simulink model "SC_TestModel"  (R2022b)
settings: Solver=VariableStepAuto  StartTime=0.0  StopTime=SimTime  RelTol=1e-3
undefined symbols (not defined in the file or in its folder): R_bal, SC_nm, SC_np, SC_ns, SC_rc, SC_rv
libraries: spsCurrentMeasurementLib x2, spsSeriesRLCBranchLib x2, spsSupercapacitorLib x1, sps_lib x1
settings Model: Creator=xuupp  LastModifiedBy=xuupp
settings DataIOCC: ReturnWorkspaceOutputs=off

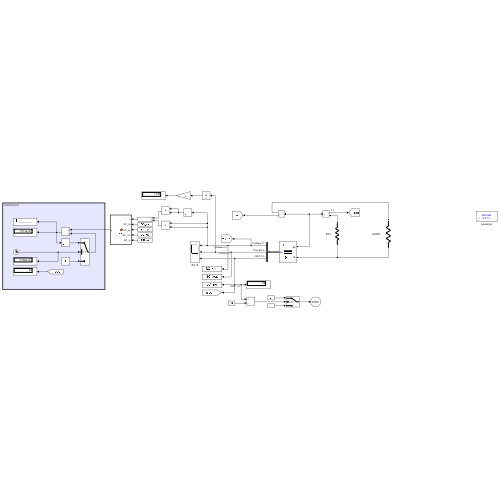
[thumbnail: Simulink's stored preview of the top-level diagram]
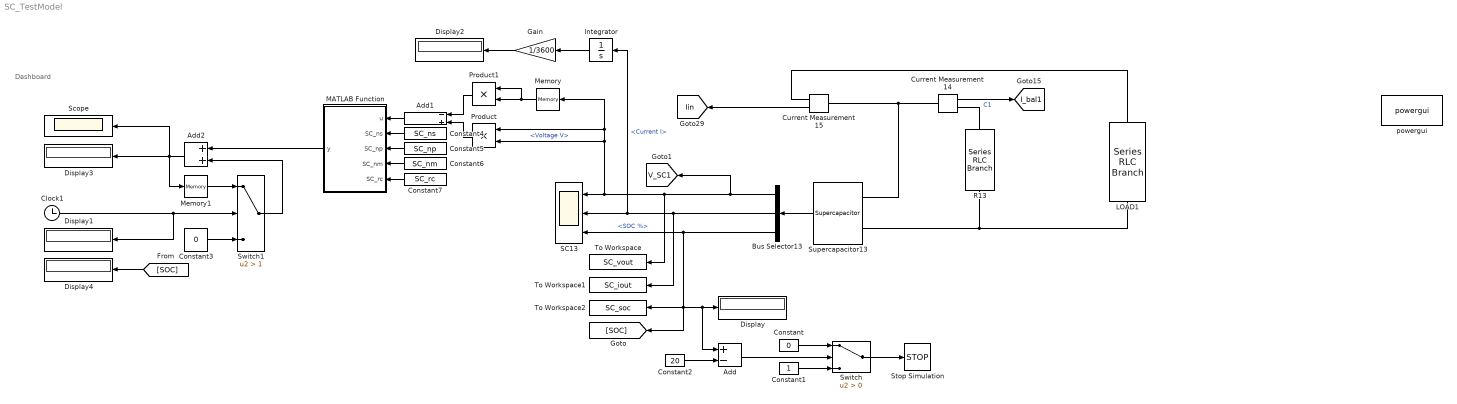
== system SC_TestModel ==
  note: Dashboard
  Add : Sum  Inputs=+-
  Add1 : Sum  Inputs=-+
  Add2 : Sum
  Bus Selector13 : BusSelector  OutputSignals=Voltage V,Current I,SOC %
  Clock1 : Clock
  Constant : Constant  Value=0
  Constant1 : Constant
  Constant2 : Constant  Value=20
  Constant3 : Constant  Value=0
  Constant4 : Constant  Value=SC_ns
  Constant5 : Constant  Value=SC_np
  Constant6 : Constant  Value=SC_nm
  Constant7 : Constant  Value=SC_rc
  Current Measurement14 : spsCurrentMeasurementLib/Current Measurement  PhasorSimulation=off  OutputType=Complex  PSBequivalent=0
  Current Measurement15 : spsCurrentMeasurementLib/Current Measurement  PhasorSimulation=off  OutputType=Complex  PSBequivalent=0
  Display{,1..4} (5 alike) : Display
  Gain : Gain  Gain=1/3600
  Integrator : Integrator
  LOAD1 : spsSeriesRLCBranchLib/Series RLC Branch  LConnTagsString=__new0  RConnTagsString=__new0  BranchType=R  Resistance=10  Inductance=1e-3  SetiL0=off  InitialCurrent=0  Capacitance=1e-5  Setx0=on  InitialVoltage=0  Measurements=Branch voltage and current
  MATLAB Function : MATLAB Function  TreatAsAtomicUnit=on
  Memory : Memory
  Memory1 : Memory
  Product : Product
  Product1 : Product
  R13 : spsSeriesRLCBranchLib/Series RLC Branch  LConnTagsString=__new0  RConnTagsString=__new0  BranchType=R  Resistance=R_bal  Inductance=1e-3  SetiL0=off  InitialCurrent=0  Capacitance=54.3e-6  Setx0=on  InitialVoltage=160  Measurements=None
  SC13 : Scope  NumInputPorts=3
  Scope : Scope
  Stop Simulation : Stop
  Supercapacitor13 : spsSupercapacitorLib/Supercapacitor  C=SC_rc  Rdc=8.9e-3  Voltage=SC_rv  Ns=N_SC_Series  Np=N_SC_Parallel  Vinit=SC_iv  Temp=25  PresetModel=off  EstParam=off  Nc=1  r=1e-9  epsilon=6.0208e-10  Ich=10  Vstern="[0.161  2.7  7.8]"  Self_dis=off  Ioc=10  Vself="[48  47.8  47.06  44.65]"  demandeplot=off  I="[10  20 100  500]"  Units=sec  Vmax=0  If=0  deltaV=0  alpha=0  sec=0
      settings: LibrarySourceBlock=sps_lib/Sources/Supercapacitor
  Switch : Switch  Criteria=u2 > Threshold  SaturateOnIntegerOverflow=off  InputSameDT=off
  Switch1 : Switch  Criteria=u2 > Threshold  Threshold=1  SaturateOnIntegerOverflow=off  InputSameDT=off
  To Workspace : ToWorkspace  VariableName=SC_vout  SampleTime=-1
  To Workspace1 : ToWorkspace  VariableName=SC_iout  SampleTime=-1
  To Workspace2 : ToWorkspace  VariableName=SC_soc  SampleTime=-1
  powergui : sps_lib/powergui  Priority=1  SimulationMode=Discrete  SampleTime=0.01  frequency=60  Iterations=50  frequencyindice=0  Pbase=100e6  ErrMax=1e-4  UnitsV=kV  UnitsW=MW  buscounter=0  FunctionMessages=off  echomessages=off  EnableUseOfTLC=off  CurrentSourceSwitches=off  DisableSnubberDevices=off  DisableRonSwitches=off  DisableVfSwitches=off  DisplayEquations=off  AutomaticDiscreteSolvers=off  SolverType=Tustin/Backward Euler (TBE)  Interpol=off  ExternalGateDelay=off  methode=off  Ts=100  x0status=blocks  SPID=on  SwTol=0  HookPort=off  NonlinearTolerance=1e-4  nMaxIteration=100  ContinueOnMaxIteration=off  RestoreLinks=warning  ResistiveCurrentMeasurement=off  Frange=[0:2:500]  Ylog=off  Xlog=on  ShowGrid=off  save=off  variable=ZData  structure=0  ZoomFFT=off  StartTime=0.0  cycles=1  DisplayStyle=1  fundamental=60  FreqAxis=off  MaxFrequency=1000  frequencyindicesteady=1  RmsSteady=1  display=off
  tag scope: I_bal1=global, Iin=global, V_SC1=global
  wires:
  Supercapacitor13/1 -> Bus Selector13/1
  Current Measurement15/1 -> [Iin]
  Current Measurement14/1 -> [I_bal1]  "C1"
  Gain/1 -> Display2/1
  Integrator/1 -> Gain/1
  Bus Selector13/1 -> To Workspace/1, Product/2, Product/1, Memory/1, SC13/1, [V_SC1]  "<Voltage V>"
  Constant2/1 -> Add/2
  Bus Selector13/2 -> To Workspace1/1, Integrator/1, SC13/2  "<Current I>"
  Constant/1 -> Switch/1
  Constant1/1 -> Switch/3
  Switch/1 -> Stop Simulation/1
  Add/1 -> Switch/2
  Bus Selector13/3 -> [SOC], Add/1, Display/1, To Workspace2/1, SC13/3  "<SOC %>"
  Memory/1 -> Product1/1, Product1/2
  Product/1 -> Add1/2
  Product1/1 -> Add1/1
  MATLAB Function/1(y) -> Add2/1
  Switch1/1 -> Add2/2
  Add2/1 -> Scope/1, Display3/1, Memory1/1
  Clock1/1 -> Display1/1, Switch1/2
  Memory1/1 -> Switch1/1
  Constant3/1 -> Switch1/3
  [SOC] -> Display4/1
  Constant4/1 -> MATLAB Function/2(SC_ns)
  Constant5/1 -> MATLAB Function/3(SC_np)
  Constant6/1 -> MATLAB Function/4(SC_nm)
  Constant7/1 -> MATLAB Function/5(SC_rc)
  Add1/1 -> MATLAB Function/1(u)
  connections:
  Current Measurement14/LConn1 -- Supercapacitor13/LConn1 -- Current Measurement15/LConn1
  R13/RConn1 -- Supercapacitor13/LConn2 -- LOAD1/RConn1
  Current Measurement14/RConn1 -- R13/LConn1
  Current Measurement15/RConn1 -- LOAD1/LConn1

== matlab function SC_TestModel/MATLAB Function ==
  data: u input; y output; SC_ns input; SC_np input; SC_nm input; SC_rc input
function y = fcn(u,SC_ns,SC_np,SC_nm,SC_rc)

y = abs(SC_ns*SC_np*SC_nm*SC_rc/2*u);
